simulink model "MainModelECU1_Limited"  (R2017b)
settings: Solver=FixedStepDiscrete  StartTime=0.0  StopTime=inf  RelTol=1e-3  EnableMultiTasking=on
undefined symbols (not defined in the file): GPTRIP1SEL, GPTRIP2SEL, Ki, Kp, r, TZ1, TZ2
libraries: canmsglib x4, c280xlib x4, c2802xlib x2, hdlsllib x1, simulink x1
settings Model: ExtModeTrigDuration=8  Creator=Teodo  LastModifiedBy=Teodo
settings OptimizationCC: DefaultUnderspecifiedDataType=single  PassReuseOutputArgsAs=Individual arguments  MaxStackSize=512
settings DebuggingCC: ParameterTunabilityLossMsg=error
settings HardwareCC: ProdBitPerChar=16  ProdBitPerInt=16  ProdBitPerPointer=32  ProdBitPerSizeT=32  ProdBitPerPtrDiffT=32  ProdLargestAtomicInteger=Integer  ProdLargestAtomicFloat=None  ProdWordSize=16  ProdLongLongMode=on  ProdHWDeviceType=Texas Instruments->C2000
settings SFSimCC: MATLABDynamicMemAlloc=off
settings RTWCC: SystemTargetFile=ert.tlc  HardwareBoard=TI Piccolo F2806x (boot from flash)  TLCOptions=-aInlineSetEventsForThisBaseRateFcn=TLC_FALSE -aSuppressMultiTaskScheduler=TLC_FALSE -aRateBasedStepFcn=1  TemplateMakefile=ert_default_tmf  GenerateReport=on  Toolchain=Texas Instruments Code Composer Studio (C2000)  IncludeHyperlinkInReport=on  LaunchReport=on  GenerateTraceInfo=on  GenerateTraceReport=on  GenerateTraceReportSl=on  GenerateTraceReportSf=on  GenerateTraceReportEml=on
settings CodeAppCC: ForceParamTrailComments=on  IgnoreCustomStorageClasses=off  OperatorAnnotations=on  SimulinkDataObjDesc=on  SFDataObjDesc=on  InsertBlockDesc=on
settings ERTTargetCC: CodeReplacementLibrary=TI C28x

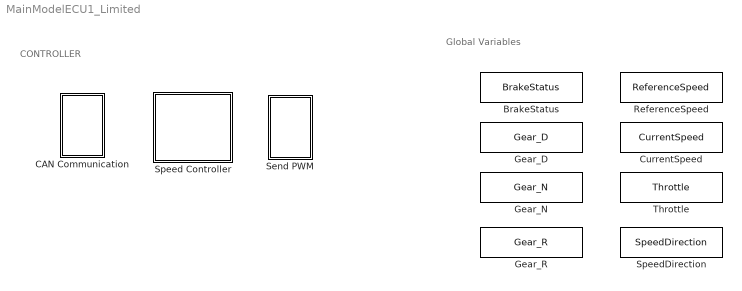
== system MainModelECU1_Limited ==
  note: CONTROLLER
  note: Global Variables
  BrakeStatus : DataStoreMemory  DataStoreName=BrakeStatus  ReadBeforeWriteMsg=warning  WriteAfterWriteMsg=warning  WriteAfterReadMsg=warning  ShowAdditionalParam=off
  CAN Communication : Subsystem
  CurrentSpeed : DataStoreMemory  DataStoreName=CurrentSpeed  ReadBeforeWriteMsg=warning  WriteAfterWriteMsg=warning  WriteAfterReadMsg=warning  ShowAdditionalParam=off
  Gear_D : DataStoreMemory  DataStoreName=Gear_D  ReadBeforeWriteMsg=warning  WriteAfterWriteMsg=warning  WriteAfterReadMsg=warning  ShowAdditionalParam=off
  Gear_N : DataStoreMemory  DataStoreName=Gear_N  ReadBeforeWriteMsg=warning  WriteAfterWriteMsg=warning  WriteAfterReadMsg=warning  ShowAdditionalParam=off
  Gear_R : DataStoreMemory  DataStoreName=Gear_R  ReadBeforeWriteMsg=warning  WriteAfterWriteMsg=warning  WriteAfterReadMsg=warning  ShowAdditionalParam=off
  ReferenceSpeed : DataStoreMemory  DataStoreName=ReferenceSpeed  ReadBeforeWriteMsg=warning  WriteAfterWriteMsg=warning  WriteAfterReadMsg=warning  ShowAdditionalParam=off
  Send PWM : Subsystem
  Speed Controller : Subsystem
  SpeedDirection : DataStoreMemory  DataStoreName=SpeedDirection  ReadBeforeWriteMsg=warning  WriteAfterWriteMsg=warning  WriteAfterReadMsg=warning  ShowAdditionalParam=off
  Throttle : DataStoreMemory  DataStoreName=Throttle  ReadBeforeWriteMsg=warning  WriteAfterWriteMsg=warning  WriteAfterReadMsg=warning  ShowAdditionalParam=off

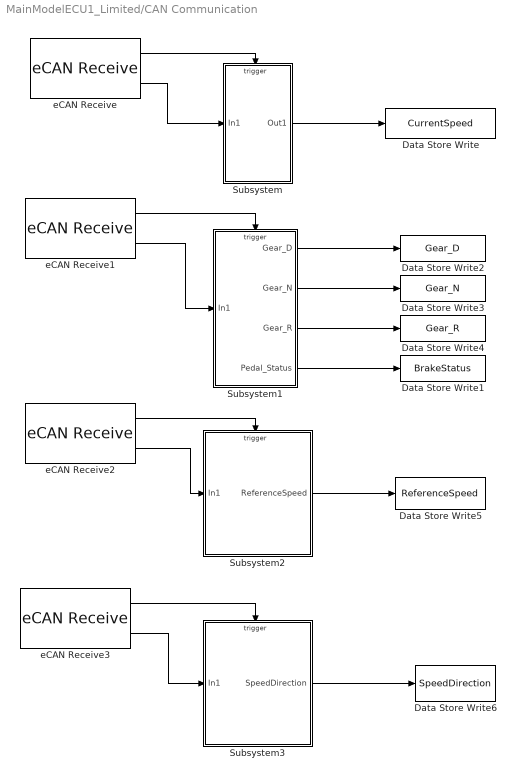
== system MainModelECU1_Limited/CAN Communication ==
  Data Store Write : DataStoreWrite  DataStoreName=CurrentSpeed
  Data Store Write1 : DataStoreWrite  DataStoreName=BrakeStatus
  Data Store Write2 : DataStoreWrite  DataStoreName=Gear_D
  Data Store Write3 : DataStoreWrite  DataStoreName=Gear_N
  Data Store Write4 : DataStoreWrite  DataStoreName=Gear_R
  Data Store Write5 : DataStoreWrite  DataStoreName=ReferenceSpeed
  Data Store Write6 : DataStoreWrite  DataStoreName=SpeedDirection
  Subsystem : Subsystem
  Subsystem1 : Subsystem
  Subsystem2 : Subsystem
  Subsystem3 : Subsystem
  eCAN Receive : c280xlib/eCAN Receive  chipFamily=C280x  useModule=eCAN_A  mailboxNo=0  messageID=1433  messageType=Standard (11-bit identifier)  sampleTime=0.01  dataType=CAN_MESSAGE_TYPE  initValue=0  outputMessageLength=off  outputMessageTimeStamp=off  postInterrupt=off  interruptLine=0
      settings: SourceProductName=Embedded Coder Support Package for Texas Instruments C2000 Processors  SourceProductBaseCode=TIC2000
  eCAN Receive1 : c280xlib/eCAN Receive  chipFamily=C280x  useModule=eCAN_A  mailboxNo=1  messageID=1435  messageType=Standard (11-bit identifier)  sampleTime=0.01  dataType=CAN_MESSAGE_TYPE  initValue=0  outputMessageLength=off  outputMessageTimeStamp=off  postInterrupt=off  interruptLine=0
      settings: SourceProductName=Embedded Coder Support Package for Texas Instruments C2000 Processors  SourceProductBaseCode=TIC2000
  eCAN Receive2 : c280xlib/eCAN Receive  chipFamily=C280x  useModule=eCAN_A  mailboxNo=2  messageID=154  messageType=Standard (11-bit identifier)  sampleTime=0.01  dataType=CAN_MESSAGE_TYPE  initValue=0  outputMessageLength=off  outputMessageTimeStamp=off  postInterrupt=off  interruptLine=0
      settings: SourceProductName=Embedded Coder Support Package for Texas Instruments C2000 Processors  SourceProductBaseCode=TIC2000
  eCAN Receive3 : c280xlib/eCAN Receive  chipFamily=C280x  useModule=eCAN_A  mailboxNo=3  messageID=415  messageType=Standard (11-bit identifier)  sampleTime=0.01  dataType=CAN_MESSAGE_TYPE  initValue=0  outputMessageLength=off  outputMessageTimeStamp=off  postInterrupt=off  interruptLine=0
      settings: SourceProductName=Embedded Coder Support Package for Texas Instruments C2000 Processors  SourceProductBaseCode=TIC2000
  wires:
  eCAN Receive/2 -> Subsystem/1(In1)
  eCAN Receive/1 -> Subsystem/Trigger
  eCAN Receive1/2 -> Subsystem1/1(In1)
  Subsystem/1(Out1) -> Data Store Write/1
  eCAN Receive1/1 -> Subsystem1/Trigger
  Subsystem2/1(ReferenceSpeed) -> Data Store Write5/1
  eCAN Receive2/1 -> Subsystem2/Trigger
  eCAN Receive2/2 -> Subsystem2/1(In1)
  Subsystem1/1(Gear_D) -> Data Store Write2/1
  Subsystem1/2(Gear_N) -> Data Store Write3/1
  Subsystem1/3(Gear_R) -> Data Store Write4/1
  Subsystem1/4(Pedal_Status) -> Data Store Write1/1
  eCAN Receive3/1 -> Subsystem3/Trigger
  eCAN Receive3/2 -> Subsystem3/1(In1)
  Subsystem3/1(SpeedDirection) -> Data Store Write6/1

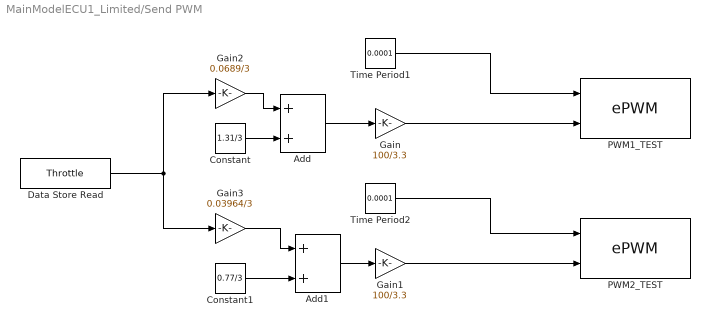
== system MainModelECU1_Limited/Send PWM ==
  Add : Sum
  Add1 : Sum
  Constant : Constant  Value=1.31/3  SampleTime=-1
  Constant1 : Constant  Value=0.77/3  SampleTime=-1
  Data Store Read : DataStoreRead  DataStoreName=Throttle
  Gain : Gain  Gain=100/3.3
  Gain1 : Gain  Gain=100/3.3
  Gain2 : Gain  Gain=0.0689/3
  Gain3 : Gain  Gain=0.03964/3
  PWM1_TEST : c2802xlib/ePWM  useModule=ePWM1  ePWMxLINKTBPRD=Not Linked  periodUnits=Seconds  timerSource=Input port  timerPeriod_clk=64000  timerPeriod_sec=0.0001  tbshadow=Counter equals to zero  countingMode=Up  phaseActiveEnable=Set counter to phase value specified via dialog  phaseDirection=Count down after sync  phaseActive=0  synchronizationEnable=off  dcaevt1Sync=off  dcbevt1Sync=off  synchronizationOption=Pass through (EPWMxSYNCI or SWFSYNC)  clockPrescale=1  HSclockPrescale=1  enswap=off  ePWMxAStatus=on  ePWMxAactionLogic1=Set  ePWMxAactionLogic2=Set  ePWMxAactionLogic3=Clear  ePWMxAactionLogic4=Set  ePWMxAactionLogic5=Do nothing  ePWMxAactionLogic6=Do nothing  ePWMxALoadMode=Load on counter equals to zero (CTR=Zero)  ePWMxACSFenable=off  ePWMxACSFvalue=Forcing disable  ePWMxASFreload=Zero  ePWMxBStatus=off  ePWMxBactionLogic1=Set  ePWMxBactionLogic2=Clear  ePWMxBactionLogic3=Do nothing  ePWMxBactionLogic4=Do nothing  ePWMxBactionLogic5=Clear  ePWMxBactionLogic6=Set  ePWMxBLoadMode=Load on counter equals to zero (CTR=Zero)  ePWMxBCSFenable=off  ePWMxBCSFvalue=Forcing disable  ePWMxBSFreload=Zero  ePWNxBOutWay=off  ePWMxLINKCMPA=Not Linked  CMPAUnits=Percentages  CMPASource=Input port  CMPAValue_per=50  CMPAValue_clk=32000  enCMPAshadow=Immediate without using shadow  ePWMxLINKCMPB=Not Linked  CMPBUnits=Percentages  CMPBSource=Specify via dialog  CMPBValue_per=50  CMPBValue_clk=32000  enCMPBshadow=Counter equals to zero  ePWMxLINKCMPC=Not Linked  CMPCUnits=Clock cycles  CMPCSource=Specify via dialog  CMPCValue_per=50  CMPCValue_clk=32000  enCMPCshadow=Counter equals to zero  ePWMxLINKCMPD=Not Linked  CMPDUnits=Clock cycles  CMPDSource=Specify via dialog  CMPDValue_per=50  CMPDValue_clk=32000  enCMPDshadow=Counter equals to zero  enableDBePWMxA=off  enableDBePWMxB=off  enhalfcycle=off  DBpolarity=Active high (AH)  DBedgeDelay=Positive  DBSource_ePWMxA=ePWMxA  DBSource_ePWMxB=ePWMxA  DBperiodSource=Specify via dialog  REDperiod=0  FEDperiod=0  adcstartModuleA=off  adcrequestEventA=First event  adcstartEventA=Digital Compare Module A Event 1 start of conversion (DCAEVT1.soc)  adcstartEventA_type2=Digital Compare Module A Event 1 start of conversion (DCAEVT1.soc)  adcstartModuleB=off  adcrequestEventB=First event  adcstartEventB=Counter equals to zero (CTR=Zero)  adcstartEventB_type2=Counter equals to zero (CTR=Zero)  intEn=on  intPrd=First event  intSel=Counter equals to period (CTR=PRD)  intSel_type2=Counter equals to zero (CTR=Zero)  hrpe=off  enHRPWM=off  HRPWM_LoadMode=Counter equals to period (CTR=PRD)  HRPWM_CTLMode=Duty or Period control mode  HRPWM_EDGMode=Both edge  hrpeb=off  enHRPWMB=off  HRPWM_LoadModeB=Counter equals to zero (CTR=ZERO)  HRPWM_CTLModeB=Duty or Period control mode  HRPWM_EDGModeB=Both edge  enSFO=on  enautoconv=on  chopperEnable=off  chopperFrequency=1  chopperFirstwidth=1  chopperDuty=12.5%  tripZonesource=Specify via dialog  tzselOSHT1=off  tzselOSHT2=off  tzselOSHT3=off  tzselOSHDCAEV1=off  tzselOSHDCBEV1=off  tzselCBC1=off  tzselCBC2=off  tzselCBC3=off  tzselCBCDCAEV2=off  tzselCBCDCBEV2=off  tzselOSHT4=off  tzselOSHT5=off  tzselOSHT6=off  tzselCBC4=off  tzselCBC5=off  tzselCBC6=off  enTzOstIntr=off  enTzCbcIntr=off  enTzDCAEVT1Intr=off  enTzDCAEVT2Intr=off  enTzDCBEVT1Intr=off  enTzDCBEVT2Intr=off  ePWMxAforced=No action  ePWMxBforced=No action  DCAEVT1forced=No action  DCBEVT1forced=No action  DCAEVT2forced=No action  DCBEVT2forced=No action  dcah=Trip Zone 1 input (TZ1)  dcal=Trip Zone 2 input (TZ2)  dcbh=Trip Zone 1 input (TZ1)  dcbl=Trip Zone 2 input (TZ2)  dcah_type2=GPTRIP1SEL/(TZ1)  dcal_type2=GPTRIP2SEL/(TZ2)  dcbh_type2=GPTRIP1SEL/(TZ1)  dcbl_type2=GPTRIP2SEL/(TZ2)  gendcaevt1=Event disabled  gendcaevt2=Event disabled  gendcbevt1=Event disabled  gendcbevt2=Event disabled  dcaevt1src=DCAEVT1 with sync  dcaevt2src=DCAEVT2 with sync  dcbevt1src=DCBEVT1 with sync  dcbevt2src=DCBEVT2 with sync  pulsesel=Counter equals to zero (CTR=Zero)  blankinv=off  blankoffset=0  blankwidth=0  evsrcsel=Filtered version of DCAEVT1 (DCAEVT1FILT)  encape=off  PwmType=C2000
      settings: SourceProductName=Embedded Coder Support Package for Texas Instruments C2000 Processors
  PWM2_TEST : c2802xlib/ePWM  useModule=ePWM2  ePWMxLINKTBPRD=Not Linked  periodUnits=Seconds  timerSource=Input port  timerPeriod_clk=64000  timerPeriod_sec=0.0001  tbshadow=Counter equals to zero  countingMode=Up  phaseActiveEnable=Set counter to phase value specified via dialog  phaseDirection=Count down after sync  phaseActive=0  synchronizationEnable=off  dcaevt1Sync=off  dcbevt1Sync=off  synchronizationOption=Pass through (EPWMxSYNCI or SWFSYNC)  clockPrescale=1  HSclockPrescale=1  enswap=off  ePWMxAStatus=on  ePWMxAactionLogic1=Set  ePWMxAactionLogic2=Set  ePWMxAactionLogic3=Clear  ePWMxAactionLogic4=Set  ePWMxAactionLogic5=Do nothing  ePWMxAactionLogic6=Do nothing  ePWMxALoadMode=Load on counter equals to zero (CTR=Zero)  ePWMxACSFenable=off  ePWMxACSFvalue=Forcing disable  ePWMxASFreload=Zero  ePWMxBStatus=off  ePWMxBactionLogic1=Set  ePWMxBactionLogic2=Clear  ePWMxBactionLogic3=Do nothing  ePWMxBactionLogic4=Do nothing  ePWMxBactionLogic5=Clear  ePWMxBactionLogic6=Set  ePWMxBLoadMode=Load on counter equals to zero (CTR=Zero)  ePWMxBCSFenable=off  ePWMxBCSFvalue=Forcing disable  ePWMxBSFreload=Zero  ePWNxBOutWay=off  ePWMxLINKCMPA=Not Linked  CMPAUnits=Percentages  CMPASource=Input port  CMPAValue_per=50  CMPAValue_clk=32000  enCMPAshadow=Immediate without using shadow  ePWMxLINKCMPB=Not Linked  CMPBUnits=Percentages  CMPBSource=Specify via dialog  CMPBValue_per=50  CMPBValue_clk=32000  enCMPBshadow=Counter equals to zero  ePWMxLINKCMPC=Not Linked  CMPCUnits=Clock cycles  CMPCSource=Specify via dialog  CMPCValue_per=50  CMPCValue_clk=32000  enCMPCshadow=Counter equals to zero  ePWMxLINKCMPD=Not Linked  CMPDUnits=Clock cycles  CMPDSource=Specify via dialog  CMPDValue_per=50  CMPDValue_clk=32000  enCMPDshadow=Counter equals to zero  enableDBePWMxA=off  enableDBePWMxB=off  enhalfcycle=off  DBpolarity=Active high (AH)  DBedgeDelay=Positive  DBSource_ePWMxA=ePWMxA  DBSource_ePWMxB=ePWMxA  DBperiodSource=Specify via dialog  REDperiod=0  FEDperiod=0  adcstartModuleA=off  adcrequestEventA=First event  adcstartEventA=Digital Compare Module A Event 1 start of conversion (DCAEVT1.soc)  adcstartEventA_type2=Digital Compare Module A Event 1 start of conversion (DCAEVT1.soc)  adcstartModuleB=off  adcrequestEventB=First event  adcstartEventB=Counter equals to zero (CTR=Zero)  adcstartEventB_type2=Counter equals to zero (CTR=Zero)  intEn=off  intPrd=First event  intSel=Counter equals to zero (CTR=Zero)  intSel_type2=Counter equals to zero (CTR=Zero)  hrpe=off  enHRPWM=off  HRPWM_LoadMode=Counter equals to period (CTR=PRD)  HRPWM_CTLMode=Duty or Period control mode  HRPWM_EDGMode=Both edge  hrpeb=off  enHRPWMB=off  HRPWM_LoadModeB=Counter equals to zero (CTR=ZERO)  HRPWM_CTLModeB=Duty or Period control mode  HRPWM_EDGModeB=Both edge  enSFO=on  enautoconv=on  chopperEnable=off  chopperFrequency=1  chopperFirstwidth=1  chopperDuty=12.5%  tripZonesource=Specify via dialog  tzselOSHT1=off  tzselOSHT2=off  tzselOSHT3=off  tzselOSHDCAEV1=off  tzselOSHDCBEV1=off  tzselCBC1=off  tzselCBC2=off  tzselCBC3=off  tzselCBCDCAEV2=off  tzselCBCDCBEV2=off  tzselOSHT4=off  tzselOSHT5=off  tzselOSHT6=off  tzselCBC4=off  tzselCBC5=off  tzselCBC6=off  enTzOstIntr=off  enTzCbcIntr=off  enTzDCAEVT1Intr=off  enTzDCAEVT2Intr=off  enTzDCBEVT1Intr=off  enTzDCBEVT2Intr=off  ePWMxAforced=No action  ePWMxBforced=No action  DCAEVT1forced=No action  DCBEVT1forced=No action  DCAEVT2forced=No action  DCBEVT2forced=No action  dcah=Trip Zone 1 input (TZ1)  dcal=Trip Zone 2 input (TZ2)  dcbh=Trip Zone 1 input (TZ1)  dcbl=Trip Zone 2 input (TZ2)  dcah_type2=GPTRIP1SEL/(TZ1)  dcal_type2=GPTRIP2SEL/(TZ2)  dcbh_type2=GPTRIP1SEL/(TZ1)  dcbl_type2=GPTRIP2SEL/(TZ2)  gendcaevt1=Event disabled  gendcaevt2=Event disabled  gendcbevt1=Event disabled  gendcbevt2=Event disabled  dcaevt1src=DCAEVT1 with sync  dcaevt2src=DCAEVT2 with sync  dcbevt1src=DCBEVT1 with sync  dcbevt2src=DCBEVT2 with sync  pulsesel=Counter equals to zero (CTR=Zero)  blankinv=off  blankoffset=0  blankwidth=0  evsrcsel=Filtered version of DCAEVT1 (DCAEVT1FILT)  encape=off  PwmType=C2000
      settings: SourceProductName=Embedded Coder Support Package for Texas Instruments C2000 Processors
  Time Period1 : Constant  Value=0.0001  SampleTime=-1
  Time Period2 : Constant  Value=0.0001  SampleTime=-1
  wires:
  Gain/1 -> PWM1_TEST/2
  Gain3/1 -> Add1/1
  Time Period1/1 -> PWM1_TEST/1
  Gain2/1 -> Add/1
  Gain1/1 -> PWM2_TEST/2
  Time Period2/1 -> PWM2_TEST/1
  Add1/1 -> Gain1/1
  Constant/1 -> Add/2
  Add/1 -> Gain/1
  Constant1/1 -> Add1/2
  Data Store Read/1 -> Gain3/1, Gain2/1

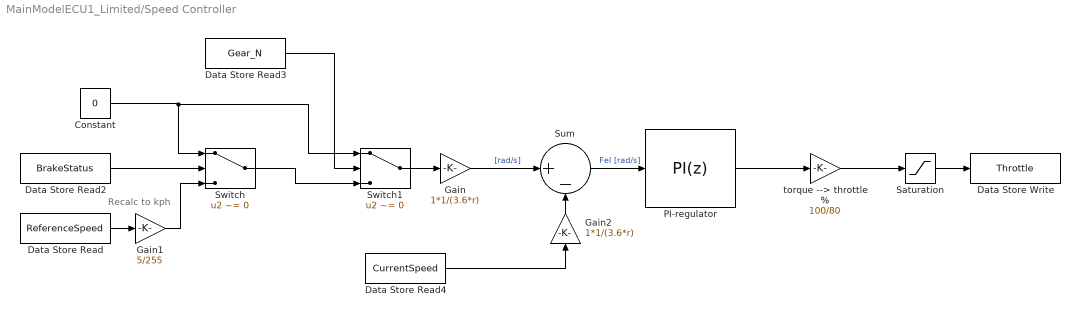
== system MainModelECU1_Limited/Speed Controller ==
  note: Recalc to kph
  Constant : Constant  Value=0  SampleTime=-1
  Data Store Read : DataStoreRead  DataStoreName=ReferenceSpeed
  Data Store Read2 : DataStoreRead  DataStoreName=BrakeStatus
  Data Store Read3 : DataStoreRead  DataStoreName=Gear_N
  Data Store Read4 : DataStoreRead  DataStoreName=CurrentSpeed
  Data Store Write : DataStoreWrite  DataStoreName=Throttle
  Gain : Gain  Gain=1*1/(3.6*r)
  Gain1 : Gain  Gain=5/255
  Gain2 : Gain  Gain=1*1/(3.6*r)
  PI-regulator : simulink/Continuous/PID Controller  Controller=PI  TimeDomain=Discrete-time  SampleTime=-1  IntegratorMethod=Trapezoidal  FilterMethod=Forward Euler  Form=Parallel  UseFilter=on  ControllerParametersSource=internal  P=Kp  I=Ki  D=0  N=100  InitialConditionSource=internal  InitialConditionForIntegrator=0  InitialConditionForFilter=0  ExternalReset=none  LimitOutput=off  UpperSaturationLimit=100  LowerSaturationLimit=0  LinearizeAsGain=on  AntiWindupMode=back-calculation  Kb=1  TrackingMode=off  Kt=1  PParamMin=[]  PParamMax=[]  IParamMin=[]  IParamMax=[]  DParamMin=[]  DParamMax=[]  NParamMin=[]  NParamMax=[]  KbParamMin=[]  KbParamMax=[]  KtParamMin=[]  KtParamMax=[]  POutMin=[]  POutMax=[]  IOutMin=[]  IOutMax=[]  DOutMin=[]  DOutMax=[]  NOutMin=[]  NOutMax=[]  KbOutMin=[]  KbOutMax=[]  KtOutMin=[]  KtOutMax=[]  IntegratorOutMin=[]  IntegratorOutMax=[]  FilterOutMin=[]  FilterOutMax=[]  SumOutMin=[]  SumOutMax=[]  SumI1OutMin=[]  SumI1OutMax=[]  SumI2OutMin=[]  SumI2OutMax=[]  SumI3OutMin=[]  SumI3OutMax=[]  SumDOutMin=[]  SumDOutMax=[]  SaturationOutMin=[]  SaturationOutMax=[]  IntegratorContinuousStateAttributes=''  IntegratorStateMustResolveToSignalObject=off  IntegratorRTWStateStorageClass=Auto  FilterContinuousStateAttributes=''  FilterStateMustResolveToSignalObject=off  FilterRTWStateStorageClass=Auto  DifferentiatorICPrevScaledInput=0  DifferentiatorOutMin=[]  DifferentiatorOutMax=[]  InitialConditionSetting=State (most efficient)  FilterDiffOutCoefMin=[]  FilterDiffOutCoefMax=[]  SumDenOutMin=[]  SumDenOutMax=[]  SumNumOutMin=[]  SumNumOutMax=[]  ReciprocalOutMin=[]  ReciprocalOutMax=[]  DivideOutMin=[]  DivideOutMax=[]  TunerSelectOption=Transfer Function Based (PID Tuner App)
  Saturation : Saturate  UpperLimit=100  LowerLimit=0
  Sum : Sum  Inputs=|+-
  Switch : Switch  Criteria=u2 ~= 0
  Switch1 : Switch  Criteria=u2 ~= 0
  torque --> throttle % : Gain  Gain=100/80
  wires:
  Data Store Read2/1 -> Switch/2
  Gain1/1 -> Switch/3
  Sum/1 -> PI-regulator/1  "Fel [rad/s]"
  Gain/1 -> Sum/1  "[rad/s]"
  PI-regulator/1 -> torque --> throttle %/1
  Gain2/1 -> Sum/2
  Data Store Read4/1 -> Gain2/1
  Data Store Read/1 -> Gain1/1
  Saturation/1 -> Data Store Write/1
  Constant/1 -> Switch1/1, Switch/1
  Switch1/1 -> Gain/1
  Data Store Read3/1 -> Switch1/2
  Switch/1 -> Switch1/3
  torque --> throttle %/1 -> Saturation/1

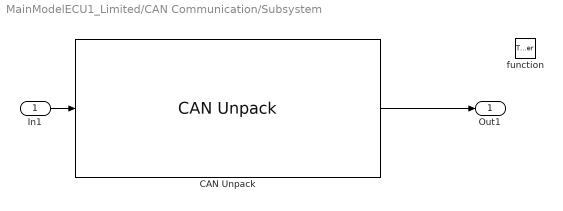
== system MainModelECU1_Limited/CAN Communication/Subsystem ==
  In1 : Inport
  function : TriggerPort  TriggerType=function-call  VariantControl=Variant
  CAN Unpack : canmsglib/CAN Unpack  CANdbFile=C:\Users\Teodo\Documents\MATLAB\Motor_Control.dbc  MsgList=CurrentSpeed  MsgName=CurrentSpeed  MsgIDType=Standard (11-bit identifier)  MsgIdentifier=1433  MsgLength=8  SignalInfo=Curr_Speed$56$16$2$2$1$0$1.000000e-02$0$-Inf$Inf$#  NSignals=1  IDPort=off  TimestampPort=off  ErrorPort=off  RemotePort=off  LengthPort=off  StatusPort=off  StartBits=str2num('[int32(56)]')  SignalSizes=str2num('[int32(16)]')  ByteOrders=str2num('[int32(2)]')  DataTypes=str2num('[int32(2)]')  MultiplexTypes=str2num('[int32(1)]')  MultiplexValues=str2num('[double(0)]')  Factors=str2num('[double(1.000000e-02)]')  Offsets=str2num('[double(0)]')  Minimums=str2num('[double(-Inf)]')  Maximums=str2num('[double(Inf)]')  ApplyMinMax=off
      settings: SourceProductName=Simulink Real-Time  SourceProductBaseCode=XP  DataFormat=CANdb specified signals
  Out1 : Outport
  wires:
  In1/1 -> CAN Unpack/1
  CAN Unpack/1 -> Out1/1

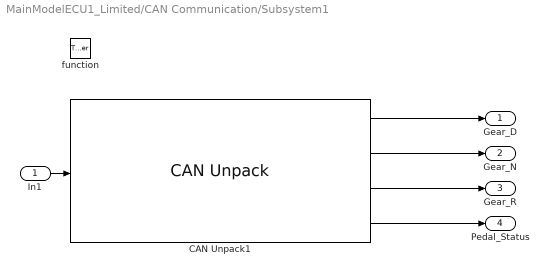
== system MainModelECU1_Limited/CAN Communication/Subsystem1 ==
  In1 : Inport
  function : TriggerPort  TriggerType=function-call  VariantControl=Variant
  CAN Unpack1 : canmsglib/CAN Unpack  CANdbFile=C:\Users\Teodo\Documents\MATLAB\Motor_Control.dbc  MsgList=Gears_Break  MsgName=Gears_Break  MsgIDType=Standard (11-bit identifier)  MsgIdentifier=1435  MsgLength=8  SignalInfo=Gear_D$7$1$1$2$1$0$1$0$-Inf$Inf$#Gear_N$5$1$1$2$1$0$1$0$-Inf$Inf$#Gear_R$3$1$1$2$1$0$1$0$-Inf$Inf$#Pedal_Status$8$1$1$2$1$0$1$0$-Inf$Inf$#  NSignals=4  IDPort=off  TimestampPort=off  ErrorPort=off  RemotePort=off  LengthPort=off  StatusPort=off  StartBits=str2num('[int32(7);int32(5);int32(3);int32(8)]')  SignalSizes=str2num('[int32(1);int32(1);int32(1);int32(1)]')  ByteOrders=str2num('[int32(1);int32(1);int32(1);int32(1)]')  DataTypes=str2num('[int32(2);int32(2);int32(2);int32(2)]')  MultiplexTypes=str2num('[int32(1);int32(1);int32(1);int32(1)]')  MultiplexValues=str2num('[double(0);double(0);double(0);double(0)]')  Factors=str2num('[double(1);double(1);double(1);double(1)]')  Offsets=str2num('[double(0);double(0);double(0);double(0)]')  Minimums=str2num('[double(-Inf);double(-Inf);double(-Inf);double(-Inf)]')  Maximums=str2num('[double(Inf);double(Inf);double(Inf);double(Inf)]')  ApplyMinMax=off
      settings: SourceProductName=Simulink Real-Time  SourceProductBaseCode=XP  DataFormat=CANdb specified signals
  Gear_D : Outport
  Gear_N : Outport  Port=2
  Gear_R : Outport  Port=3
  Pedal_Status : Outport  Port=4
  wires:
  In1/1 -> CAN Unpack1/1
  CAN Unpack1/2 -> Gear_N/1
  CAN Unpack1/4 -> Pedal_Status/1
  CAN Unpack1/3 -> Gear_R/1
  CAN Unpack1/1 -> Gear_D/1

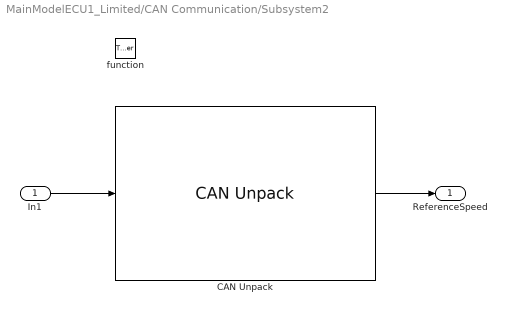
== system MainModelECU1_Limited/CAN Communication/Subsystem2 ==
  In1 : Inport
  function : TriggerPort  TriggerType=function-call  VariantControl=Variant
  CAN Unpack : canmsglib/CAN Unpack  CANdbFile=C:\Users\Teodo\Documents\MATLAB\Motor_Control.dbc  MsgList=ReferenceSpeed  MsgName=ReferenceSpeed  MsgIDType=Standard (11-bit identifier)  MsgIdentifier=154  MsgLength=8  SignalInfo=Ref_Speed$0$8$1$2$1$0$1$0$-Inf$Inf$#  NSignals=1  IDPort=off  TimestampPort=off  ErrorPort=off  RemotePort=off  LengthPort=off  StatusPort=off  StartBits=str2num('[int32(0)]')  SignalSizes=str2num('[int32(8)]')  ByteOrders=str2num('[int32(1)]')  DataTypes=str2num('[int32(2)]')  MultiplexTypes=str2num('[int32(1)]')  MultiplexValues=str2num('[double(0)]')  Factors=str2num('[double(1)]')  Offsets=str2num('[double(0)]')  Minimums=str2num('[double(-Inf)]')  Maximums=str2num('[double(Inf)]')  ApplyMinMax=off
      settings: SourceProductName=Simulink Real-Time  SourceProductBaseCode=XP  DataFormat=CANdb specified signals
  ReferenceSpeed : Outport
  wires:
  In1/1 -> CAN Unpack/1
  CAN Unpack/1 -> ReferenceSpeed/1

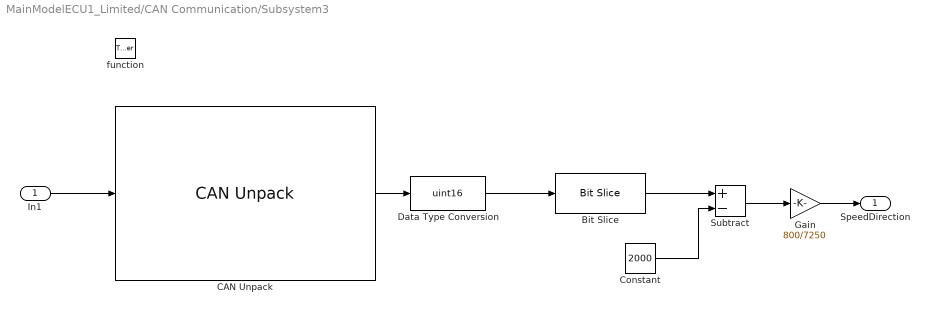
== system MainModelECU1_Limited/CAN Communication/Subsystem3 ==
  In1 : Inport
  function : TriggerPort  TriggerType=function-call  VariantControl=Variant
  Bit Slice : hdlsllib/Logic and Bit Operations/Bit Slice  lidx=15  ridx=4
  CAN Unpack : canmsglib/CAN Unpack  CANdbFile=C:\Users\Teodo\Documents\MATLAB\Motor_Control.dbc  MsgList=Speed_Dir  MsgName=Speed_Dir  MsgIDType=Standard (11-bit identifier)  MsgIdentifier=415  MsgLength=8  SignalInfo=SpeedDir$24$16$2$2$1$0$1$0$-Inf$Inf$#  NSignals=1  IDPort=off  TimestampPort=off  ErrorPort=off  RemotePort=off  LengthPort=off  StatusPort=off  StartBits=str2num('[int32(24)]')  SignalSizes=str2num('[int32(16)]')  ByteOrders=str2num('[int32(2)]')  DataTypes=str2num('[int32(2)]')  MultiplexTypes=str2num('[int32(1)]')  MultiplexValues=str2num('[double(0)]')  Factors=str2num('[double(1)]')  Offsets=str2num('[double(0)]')  Minimums=str2num('[double(-Inf)]')  Maximums=str2num('[double(Inf)]')  ApplyMinMax=off
      settings: SourceProductName=Simulink Real-Time  SourceProductBaseCode=XP  DataFormat=CANdb specified signals
  Constant : Constant  Value=2000
  Data Type Conversion : DataTypeConversion  OutDataTypeStr=uint16
  Gain : Gain  Gain=800/7250
  Subtract : Sum  Inputs=+-
  SpeedDirection : Outport
  wires:
  In1/1 -> CAN Unpack/1
  CAN Unpack/1 -> Data Type Conversion/1
  Data Type Conversion/1 -> Bit Slice/1
  Constant/1 -> Subtract/2
  Bit Slice/1 -> Subtract/1
  Subtract/1 -> Gain/1
  Gain/1 -> SpeedDirection/1
